simulink model "micro_hydro_with_elc"  (R2018a)
settings: Solver=ode23tb  StartTime=0.0  StopTime=4  FixedStep=1e-6  RelTol=1e-3
libraries: powerlib x37, powerlib_meascontrol x9, simulink x1, sps_avr x1, spsHTGModel x1
settings Model: SimulationMode=accelerator  Creator=deep  LastModifiedBy=Electrical
settings SolverCC: AlgebraicLoopSolver=LineSearch
settings OptimizationCC: EfficientMapNaN2IntZero=off
settings HardwareCC: TargetBitPerPointer=64  TargetBitPerSizeT=64  TargetBitPerPtrDiffT=64  TargetLongLongMode=on  TargetIntDivRoundTo=Zero  TargetEndianess=LittleEndian  TargetWordSize=64  TargetHWDeviceType=MATLAB Host  ProdEqTarget=off
settings SFSimCC: SimUseLocalCustomCode=on
settings RTWCC: RTWUseLocalCustomCode=on
settings CodeAppCC: MaxIdLength=128
settings GRTTargetCC: TargetLangStandard=C89/C90 (ANSI)  CombineOutputUpdateFcns=off  GRTInterface=on

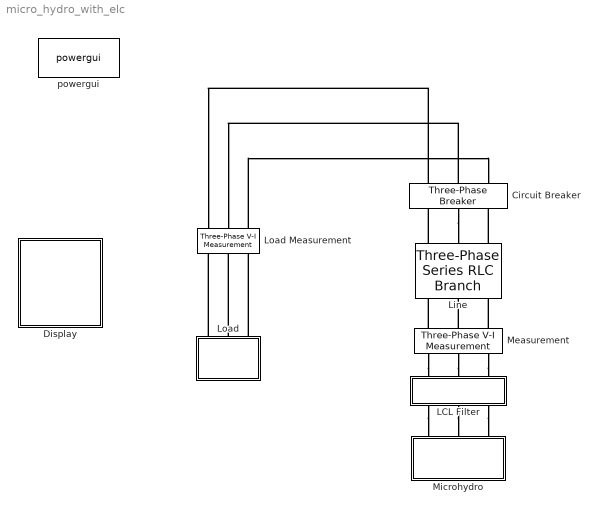
== system micro_hydro_with_elc ==
  Circuit Breaker : powerlib/Elements/Three-Phase Breaker  InitialState=open  SwitchA=on  SwitchB=on  SwitchC=on  SwitchTimes=[0.5 4]  External=off  BreakerResistance=0.00001  SnubberResistance=500000  SnubberCapacitance=inf  Measurements=None
  Display : Subsystem
  LCL Filter : Subsystem  mask{L=0.5e-3, C=100e-6}
      mask prompts: L "Inductance(L)"; C "Capacitance(C)"
  Line : powerlib/Elements/Three-Phase Series RLC Branch  LConnTagsString=A|B|C  RConnTagsString=A|B|C  BranchType=RL  Resistance=1  Inductance=0.0125  Capacitance=0  Measurements=None
  Load : Subsystem
  Load Measurement : powerlib/Measurements/Three-Phase V-I Measurement  VoltageMeasurement=phase-to-ground  SetLabelV=on  LabelV=Vload  Vpu=off  VpuLL=off  CurrentMeasurement=yes  SetLabelI=on  LabelI=Iload  Ipu=off  Pbase=100e6  Vbase=500e3  OutputType=Complex  PhasorSimulation=off  PSBequivalent=0
  Measurement : powerlib/Measurements/Three-Phase V-I Measurement  VoltageMeasurement=phase-to-ground  SetLabelV=on  LabelV=Vgrid  Vpu=off  VpuLL=off  CurrentMeasurement=yes  SetLabelI=on  LabelI=Igrid  Ipu=off  Pbase=100e6  Vbase=500e3  OutputType=Complex  PhasorSimulation=off  PSBequivalent=0
  Microhydro : Subsystem
  powergui : powerlib/powergui  Priority=1  SimulationMode=Discrete  SampleTime=1e-6  frequency=60  Iterations=50  frequencyindice=0  Pbase=100e6  ErrMax=1e-4  UnitsV=kV  UnitsW=MW  buscounter=0  FunctionMessages=off  echomessages=off  EnableUseOfTLC=off  CurrentSourceSwitches=off  DisableSnubberDevices=off  DisableRonSwitches=off  DisableVfSwitches=off  DisplayEquations=off  SolverType=Tustin/Backward Euler (TBE)  Interpol=off  ExternalGateDelay=off  methode=off  Ts=100  x0status=zero  SPID=off  SwTol=0  HookPort=off  RestoreLinks=warning  ResistiveCurrentMeasurement=off  Frange=[0:2:500]  Ylog=off  Xlog=on  ShowGrid=off  save=off  variable=ZData  structure=logsout  ZoomFFT=off  StartTime=0.0  cycles=1  DisplayStyle=1  fundamental=60  FreqAxis=off  MaxFrequency=1000  frequencyindicesteady=1  RmsSteady=1  display=off
  connections:
  Circuit Breaker/RConn1 -- Load Measurement/LConn1
  Load Measurement/LConn3 -- Circuit Breaker/RConn3
  LCL Filter/LConn2 -- Microhydro/RConn2
  LCL Filter/LConn3 -- Microhydro/RConn3
  LCL Filter/LConn1 -- Microhydro/RConn1
  Circuit Breaker/RConn2 -- Load Measurement/LConn2
  Line/RConn1 -- Circuit Breaker/LConn1
  Circuit Breaker/LConn2 -- Line/RConn2
  Line/RConn3 -- Circuit Breaker/LConn3
  Measurement/RConn1 -- Line/LConn1
  Measurement/RConn2 -- Line/LConn2
  Measurement/RConn3 -- Line/LConn3
  Measurement/LConn1 -- LCL Filter/RConn1
  Measurement/LConn2 -- LCL Filter/RConn2
  Measurement/LConn3 -- LCL Filter/RConn3
  Load/LConn1 -- Load Measurement/RConn1
  Load/LConn2 -- Load Measurement/RConn2
  Load/LConn3 -- Load Measurement/RConn3

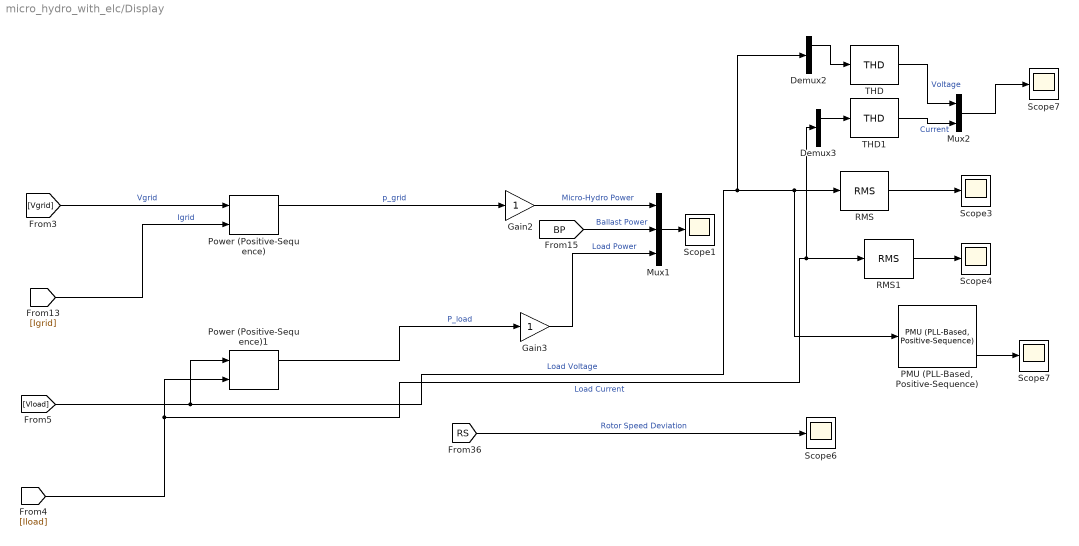
== system micro_hydro_with_elc/Display ==
  Demux2 : Demux  Outputs=3
  Demux3 : Demux  Outputs=3
  Gain2 : Gain
  Gain3 : Gain
  Mux1 : Mux  Inputs=3
  Mux2 : Mux  Inputs=2
  "PMU (PLL-Based, Positive-Sequence)" : powerlib_meascontrol/Measurements/PMU (PLL-Based, Positive-Sequence)  nominalFrequency=50  samplingRate=64  reportingFactor=1
      settings: SourceProductName=Simscape Power Systems  SourceProductBaseCode=PS
  Power (Positive-Sequence) : powerlib_meascontrol/Measurements/Power (Positive-Sequence)  Freq=50  Vinit=[0, 0]  Iinit=[0, 0]  Ts=0
      settings: SourceProductName=Simscape Power Systems  SourceProductBaseCode=PS
  Power (Positive-Sequence)1 : powerlib_meascontrol/Measurements/Power (Positive-Sequence)  Freq=50  Vinit=[0, 0]  Iinit=[0, 0]  Ts=0
      settings: SourceProductName=Simscape Power Systems  SourceProductBaseCode=PS
  RMS : powerlib_meascontrol/Measurements/RMS  TrueRMS=on  Freq=50  RMSInit=0  Ts=0
  RMS1 : powerlib_meascontrol/Measurements/RMS  TrueRMS=on  Freq=50  RMSInit=0  Ts=0
  Scope{1,3..4,6..7} (5 alike) : Scope
  "Scope7 " : Scope
  THD : powerlib_meascontrol/Measurements/THD  Freq=50  Ts=0
  THD1 : powerlib_meascontrol/Measurements/THD  Freq=50  Ts=0
  wires:
  Power (Positive-Sequence)/1 -> Gain2/1  "p_grid"
  [Vgrid] -> Power (Positive-Sequence)/1  "Vgrid"
  [Iload] -> Power (Positive-Sequence)1/2, Demux3/1, RMS1/1  "Load Current"
  Power (Positive-Sequence)1/1 -> Gain3/1  "P_load"
  [RS] -> Scope6/1  "Rotor Speed Deviation"
  [Vload] -> Power (Positive-Sequence)1/1, Demux2/1, "PMU (PLL-Based, Positive-Sequence)"/1, RMS/1  "Load Voltage"
  Mux1/1 -> Scope1/1
  RMS/1 -> Scope3/1
  RMS1/1 -> Scope4/1
  "PMU (PLL-Based, Positive-Sequence)"/3 -> Scope7/1
  Demux2/1 -> THD/1
  Demux3/1 -> THD1/1
  THD/1 -> Mux2/1  "Voltage"
  THD1/1 -> Mux2/2  "Current"
  Mux2/1 -> "Scope7 "/1
  Gain2/1 -> Mux1/1  "Micro-Hydro Power"
  [BP] -> Mux1/2  "Ballast Power"
  Gain3/1 -> Mux1/3  "Load Power"
  [Igrid] -> Power (Positive-Sequence)/2  "Igrid"

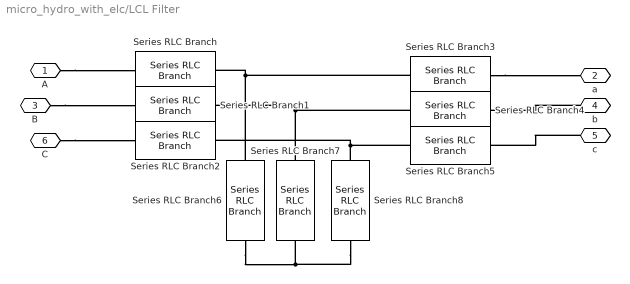
== system micro_hydro_with_elc/LCL Filter ==
  Series RLC Branch{,1..5} (6 alike) : powerlib/Elements/Series RLC Branch  LConnTagsString=__new0  RConnTagsString=__new0  BranchType=L  Resistance=1  Inductance=L  SetiL0=off  InitialCurrent=0  Capacitance=1e-6  Setx0=off  InitialVoltage=0  Measurements=None
  Series RLC Branch6 : powerlib/Elements/Series RLC Branch  LConnTagsString=__new0  RConnTagsString=__new0  BranchType=C  Resistance=1  Inductance=0.5e-3  SetiL0=off  InitialCurrent=0  Capacitance=C  Setx0=off  InitialVoltage=0  Measurements=None
  Series RLC Branch7 : powerlib/Elements/Series RLC Branch  LConnTagsString=__new0  RConnTagsString=__new0  BranchType=C  Resistance=1  Inductance=0.5e-3  SetiL0=off  InitialCurrent=0  Capacitance=C  Setx0=off  InitialVoltage=0  Measurements=None
  Series RLC Branch8 : powerlib/Elements/Series RLC Branch  LConnTagsString=__new0  RConnTagsString=__new0  BranchType=C  Resistance=1  Inductance=0.5e-3  SetiL0=off  InitialCurrent=0  Capacitance=C  Setx0=off  InitialVoltage=0  Measurements=None
  A : PMIOPort  Side=Left
  a : PMIOPort  Port=2  Side=Right
  B : PMIOPort  Port=3  Side=Left
  b : PMIOPort  Port=4  Side=Right
  c : PMIOPort  Port=5  Side=Right
  C : PMIOPort  Port=6  Side=Left
  connections:
  C/RConn1 -- Series RLC Branch2/LConn1
  Series RLC Branch3/LConn1 -- Series RLC Branch/RConn1 -- Series RLC Branch6/LConn1
  Series RLC Branch3/RConn1 -- a/RConn1
  Series RLC Branch6/RConn1 -- Series RLC Branch8/RConn1 -- Series RLC Branch7/RConn1
  Series RLC Branch5/LConn1 -- Series RLC Branch2/RConn1 -- Series RLC Branch8/LConn1
  Series RLC Branch4/LConn1 -- Series RLC Branch1/RConn1 -- Series RLC Branch7/LConn1
  c/RConn1 -- Series RLC Branch5/RConn1
  A/RConn1 -- Series RLC Branch/LConn1
  B/RConn1 -- Series RLC Branch1/LConn1
  b/RConn1 -- Series RLC Branch4/RConn1

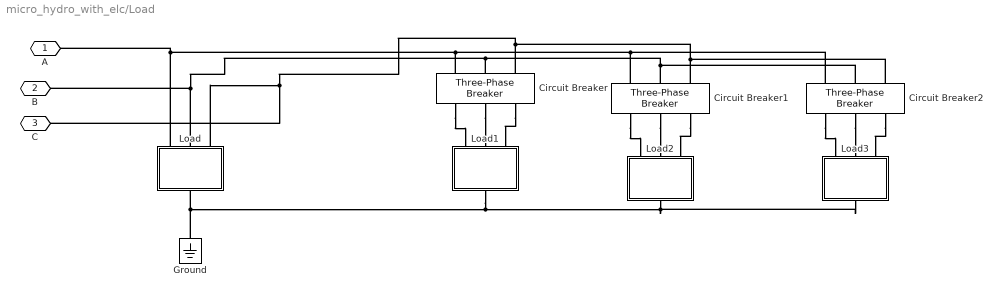
== system micro_hydro_with_elc/Load ==
  Circuit Breaker : powerlib/Elements/Three-Phase Breaker  InitialState=open  SwitchA=on  SwitchB=on  SwitchC=on  SwitchTimes=[1.5 4]  External=off  BreakerResistance=0.00001  SnubberResistance=500000  SnubberCapacitance=inf  Measurements=None
  Circuit Breaker1 : powerlib/Elements/Three-Phase Breaker  InitialState=open  SwitchA=on  SwitchB=on  SwitchC=on  SwitchTimes=[2.5 4]  External=off  BreakerResistance=0.00001  SnubberResistance=500000  SnubberCapacitance=inf  Measurements=None
  Circuit Breaker2 : powerlib/Elements/Three-Phase Breaker  InitialState=open  SwitchA=on  SwitchB=on  SwitchC=on  SwitchTimes=[3.5 4]  External=off  BreakerResistance=0.00001  SnubberResistance=500000  SnubberCapacitance=inf  Measurements=None
  Ground : powerlib/Elements/Ground  LConnTagsString=a
  Load : Subsystem  mask{R=100}
      mask prompts: R "Load Resistance"
      mask DialogControl DescTextVar Prompt: Load in terms of Resistance
  Load1 : Subsystem  mask{R=100}
      mask prompts: R "Load Resistance"
      mask DialogControl DescTextVar Prompt: Load in terms of Resistance
  Load2 : Subsystem  mask{R=100}
      mask prompts: R "Load Resistance"
      mask DialogControl DescTextVar Prompt: Load in terms of Resistance
  Load3 : Subsystem  mask{R=100}
      mask prompts: R "Load Resistance"
      mask DialogControl DescTextVar Prompt: Load in terms of Resistance
  A : PMIOPort  Side=Left
  B : PMIOPort  Port=2  Side=Left
  C : PMIOPort  Port=3  Side=Left
  connections:
  Ground/LConn1 -- Load3/RConn1 -- Load2/RConn1 -- Load1/RConn1 -- Load/RConn1
  Load/LConn1 -- Circuit Breaker2/RConn1 -- Circuit Breaker1/RConn1 -- Circuit Breaker/RConn1 -- A/RConn1
  Load/LConn2 -- Circuit Breaker2/RConn2 -- Circuit Breaker1/RConn2 -- Circuit Breaker/RConn2 -- B/RConn1
  Load/LConn3 -- Circuit Breaker2/RConn3 -- Circuit Breaker1/RConn3 -- Circuit Breaker/RConn3 -- C/RConn1
  Circuit Breaker/LConn2 -- Load1/LConn2
  Circuit Breaker/LConn1 -- Load1/LConn1
  Circuit Breaker/LConn3 -- Load1/LConn3
  Circuit Breaker1/LConn2 -- Load2/LConn2
  Circuit Breaker1/LConn1 -- Load2/LConn1
  Circuit Breaker1/LConn3 -- Load2/LConn3
  Circuit Breaker2/LConn2 -- Load3/LConn2
  Circuit Breaker2/LConn1 -- Load3/LConn1
  Circuit Breaker2/LConn3 -- Load3/LConn3

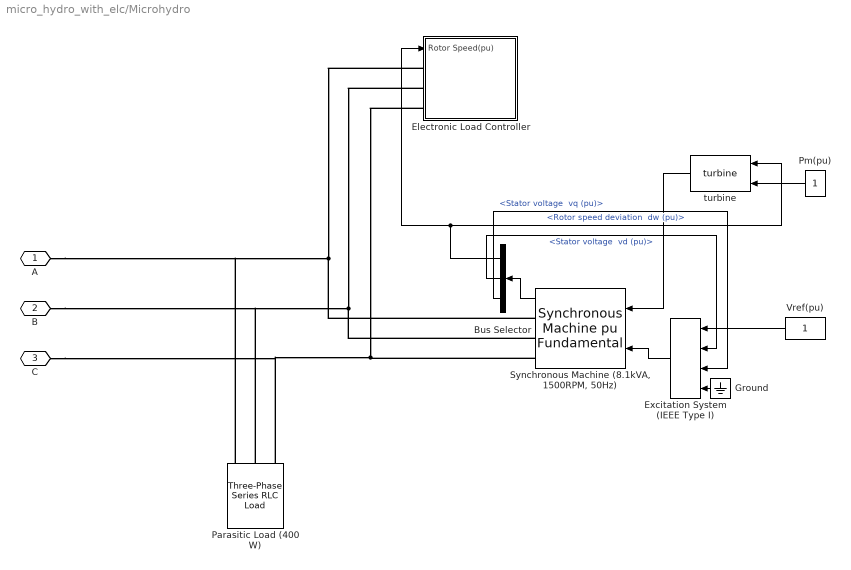
== system micro_hydro_with_elc/Microhydro ==
  Bus Selector : BusSelector  OutputSignals="Mechanical.Rotor speed deviation  dw (pu),dq0 components.Stator voltage  vd (pu),dq0 components.Stator voltage  vq (pu)"
  Electronic Load Controller : Subsystem
  Excitation System (IEEE Type I) : sps_avr/Excitation System  tr=20e-3  reg=[ 300, 0.001 ]  exc=[ 1, 0 ]  tgr=[ 0, 0 ]  damp=[ 0.001, 0.1 ]  sat=[ 0, 0 ]  lim=[ -11.5, 11.5, 0 ]  v0="[1.0  1.28]"
      settings: SourceProductName=Simscape Power Systems  SourceProductBaseCode=PS
  Ground : Ground
  Parasitic Load (400 W) : powerlib/Elements/Three-Phase Series RLC Load  LConnTagsString=A|B|C  Configuration=Y (grounded)  NominalVoltage=400  Vabc=[1e3 1e3 1e3]  Vabcp=[1e3 1e3 1e3]  NominalFrequency=50  UnbalancedPower=off  ActivePower=400  InductivePower=0  CapacitivePower=0  Pabc=[10e3 9e3 11e3]  QLabc=[100 90 110]  QCabc=[100 90 110]  Pabcp=[10e3 9e3 11e3]  QLabcp=[100 90 110]  QCabcp=[100 90 110]  Measurements=None  LoadType=constant Z
  Pm(pu) : Constant  SampleTime=-1
  "Synchronous Machine (8.1kVA, 1500RPM, 50Hz)" : powerlib/Machines/Synchronous Machine pu Fundamental  PresetModel=01: 50Hz 400V 8.1kVA 1500RPM  MechanicalLoad=Mechanical power Pm  ShowDetailedParameters=on  RotorType=Salient-pole  Units=per unit fundamental parameters  MeasurementBus=off  NominalParameters=[8100 400 50]  Stator=[0.08201 0.072 1.728 0.823]  Field=[0.06117 0.1801]  Dampers2=[0.0652, 0.5134, 0.0287, 0.2553, 7.765e-3, 0.9167 ]  Dampers1=[0.1591 0.1166 0.2416 0.1615]  Mechanical=[0.1406 0.02742 2]  PolePairs=2  InitialConditions="[ 0  0  0  0  0  0  -120  -240  1 ]"  SetSaturation=off  Saturation=[0.6404,0.7127,0.8441,0.9214,0.9956,1.082,1.19,1.316,1.457;0.7,0.7698,0.8872,0.9466,0.9969,1.046,1.1,1.151,1.201]  LoadFlowParameters=[1,0,0,0,0]  TsPowergui=0  TsBlock=-1  IterativeModel=Trapezoidal non iterative  IterativeDiscreteModel=Trapezoidal non iterative  BusType=PV  Pref=8100  Qref=0  Qmin=-inf  Qmax=inf  PLF=0  QLF=0
      settings: SourceProductName=Simscape Power Systems  SourceProductBaseCode=PS
  Vref(pu) : Constant  SampleTime=-1
  turbine : spsHTGModel/Discrete/turbine  SystemSampleTime=-1
      link override Gain2: Gain=1/1
      link override beta: Gain=1
      link override position: InitialCondition=1
      link override turbine gain: Gain=1
  A : PMIOPort  Side=Right
  B : PMIOPort  Port=2  Side=Right
  C : PMIOPort  Port=3  Side=Right
  wires:
  Bus Selector/1 -> turbine/1, Electronic Load Controller/1(Rotor Speed(pu))  "<Rotor speed deviation  dw (pu)>"
  "Synchronous Machine (8.1kVA, 1500RPM, 50Hz)"/1 -> Bus Selector/1
  Excitation System (IEEE Type I)/1 -> "Synchronous Machine (8.1kVA, 1500RPM, 50Hz)"/2
  Bus Selector/2 -> Excitation System (IEEE Type I)/2  "<Stator voltage  vd (pu)>"
  Bus Selector/3 -> Excitation System (IEEE Type I)/3  "<Stator voltage  vq (pu)>"
  Ground/1 -> Excitation System (IEEE Type I)/4
  Pm(pu)/1 -> turbine/2
  turbine/1 -> "Synchronous Machine (8.1kVA, 1500RPM, 50Hz)"/1
  Vref(pu)/1 -> Excitation System (IEEE Type I)/1
  connections:
  Electronic Load Controller/LConn2 -- B/RConn1 -- Parasitic Load (400 W)/LConn2 -- "Synchronous Machine (8.1kVA, 1500RPM, 50Hz)"/RConn2
  Electronic Load Controller/LConn1 -- A/RConn1 -- Parasitic Load (400 W)/LConn1 -- "Synchronous Machine (8.1kVA, 1500RPM, 50Hz)"/RConn1
  Electronic Load Controller/LConn3 -- Parasitic Load (400 W)/LConn3 -- C/RConn1 -- "Synchronous Machine (8.1kVA, 1500RPM, 50Hz)"/RConn3

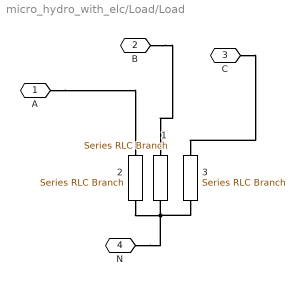
== system micro_hydro_with_elc/Load/Load ==
  1 : powerlib/Elements/Series RLC Branch  LConnTagsString=__new0  RConnTagsString=__new0  BranchType=R  Resistance=R  Inductance=10e-3  SetiL0=off  InitialCurrent=0  Capacitance=1e-6  Setx0=off  InitialVoltage=0  Measurements=None
  2 : powerlib/Elements/Series RLC Branch  LConnTagsString=__new0  RConnTagsString=__new0  BranchType=R  Resistance=R  Inductance=10e-3  SetiL0=off  InitialCurrent=0  Capacitance=1e-6  Setx0=off  InitialVoltage=0  Measurements=None
  3 : powerlib/Elements/Series RLC Branch  LConnTagsString=__new0  RConnTagsString=__new0  BranchType=R  Resistance=R  Inductance=10e-3  SetiL0=off  InitialCurrent=0  Capacitance=1e-6  Setx0=off  InitialVoltage=0  Measurements=None
  A : PMIOPort  Side=Left
  B : PMIOPort  Port=2  Side=Left
  C : PMIOPort  Port=3  Side=Left
  N : PMIOPort  Port=4  Side=Right
  connections:
  A/RConn1 -- 2/LConn1
  B/RConn1 -- 1/LConn1
  C/RConn1 -- 3/LConn1
  1/RConn1 -- 3/RConn1 -- N/RConn1 -- 2/RConn1

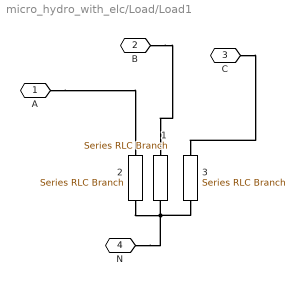
== system micro_hydro_with_elc/Load/Load1 ==
  1 : powerlib/Elements/Series RLC Branch  LConnTagsString=__new0  RConnTagsString=__new0  BranchType=R  Resistance=R  Inductance=10e-3  SetiL0=off  InitialCurrent=0  Capacitance=1e-6  Setx0=off  InitialVoltage=0  Measurements=None
  2 : powerlib/Elements/Series RLC Branch  LConnTagsString=__new0  RConnTagsString=__new0  BranchType=R  Resistance=R  Inductance=10e-3  SetiL0=off  InitialCurrent=0  Capacitance=1e-6  Setx0=off  InitialVoltage=0  Measurements=None
  3 : powerlib/Elements/Series RLC Branch  LConnTagsString=__new0  RConnTagsString=__new0  BranchType=R  Resistance=R  Inductance=10e-3  SetiL0=off  InitialCurrent=0  Capacitance=1e-6  Setx0=off  InitialVoltage=0  Measurements=None
  A : PMIOPort  Side=Left
  B : PMIOPort  Port=2  Side=Left
  C : PMIOPort  Port=3  Side=Left
  N : PMIOPort  Port=4  Side=Right
  connections:
  A/RConn1 -- 2/LConn1
  B/RConn1 -- 1/LConn1
  C/RConn1 -- 3/LConn1
  1/RConn1 -- 3/RConn1 -- N/RConn1 -- 2/RConn1

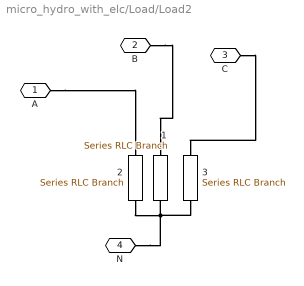
== system micro_hydro_with_elc/Load/Load2 ==
  1 : powerlib/Elements/Series RLC Branch  LConnTagsString=__new0  RConnTagsString=__new0  BranchType=R  Resistance=R  Inductance=10e-3  SetiL0=off  InitialCurrent=0  Capacitance=1e-6  Setx0=off  InitialVoltage=0  Measurements=None
  2 : powerlib/Elements/Series RLC Branch  LConnTagsString=__new0  RConnTagsString=__new0  BranchType=R  Resistance=R  Inductance=10e-3  SetiL0=off  InitialCurrent=0  Capacitance=1e-6  Setx0=off  InitialVoltage=0  Measurements=None
  3 : powerlib/Elements/Series RLC Branch  LConnTagsString=__new0  RConnTagsString=__new0  BranchType=R  Resistance=R  Inductance=10e-3  SetiL0=off  InitialCurrent=0  Capacitance=1e-6  Setx0=off  InitialVoltage=0  Measurements=None
  A : PMIOPort  Side=Left
  B : PMIOPort  Port=2  Side=Left
  C : PMIOPort  Port=3  Side=Left
  N : PMIOPort  Port=4  Side=Right
  connections:
  A/RConn1 -- 2/LConn1
  B/RConn1 -- 1/LConn1
  C/RConn1 -- 3/LConn1
  1/RConn1 -- 3/RConn1 -- N/RConn1 -- 2/RConn1

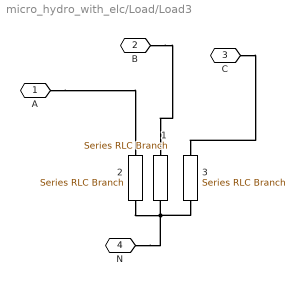
== system micro_hydro_with_elc/Load/Load3 ==
  1 : powerlib/Elements/Series RLC Branch  LConnTagsString=__new0  RConnTagsString=__new0  BranchType=R  Resistance=R  Inductance=10e-3  SetiL0=off  InitialCurrent=0  Capacitance=1e-6  Setx0=off  InitialVoltage=0  Measurements=None
  2 : powerlib/Elements/Series RLC Branch  LConnTagsString=__new0  RConnTagsString=__new0  BranchType=R  Resistance=R  Inductance=10e-3  SetiL0=off  InitialCurrent=0  Capacitance=1e-6  Setx0=off  InitialVoltage=0  Measurements=None
  3 : powerlib/Elements/Series RLC Branch  LConnTagsString=__new0  RConnTagsString=__new0  BranchType=R  Resistance=R  Inductance=10e-3  SetiL0=off  InitialCurrent=0  Capacitance=1e-6  Setx0=off  InitialVoltage=0  Measurements=None
  A : PMIOPort  Side=Left
  B : PMIOPort  Port=2  Side=Left
  C : PMIOPort  Port=3  Side=Left
  N : PMIOPort  Port=4  Side=Right
  connections:
  A/RConn1 -- 2/LConn1
  B/RConn1 -- 1/LConn1
  C/RConn1 -- 3/LConn1
  1/RConn1 -- 3/RConn1 -- N/RConn1 -- 2/RConn1

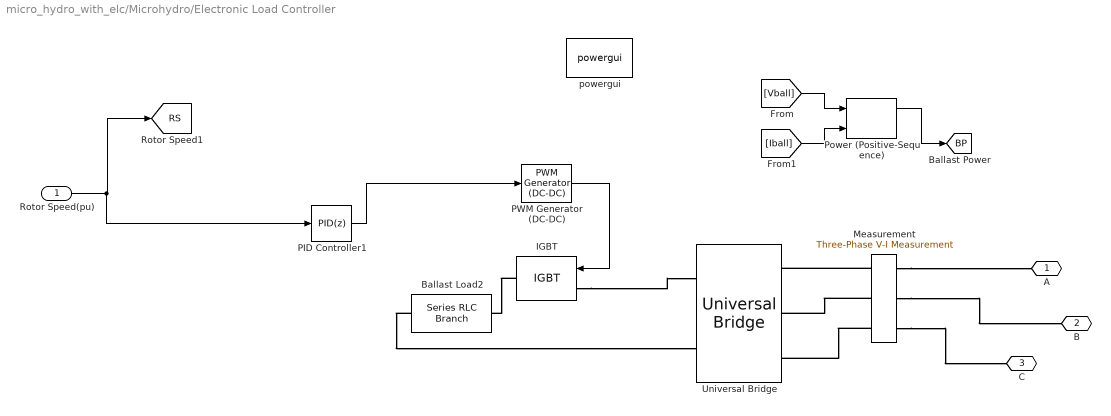
== system micro_hydro_with_elc/Microhydro/Electronic Load Controller ==
  Rotor Speed(pu) : Inport
  Ballast Load2 : powerlib/Elements/Series RLC Branch  LConnTagsString=__new0  RConnTagsString=__new0  BranchType=R  Resistance=10  Inductance=10e-3  SetiL0=off  InitialCurrent=0  Capacitance=1e-6  Setx0=off  InitialVoltage=0  Measurements=None
  IGBT : powerlib/Power Electronics/IGBT  Ron=0.001  Lon=0  Vf=1  Tf=1e-6  Tt=2e-6  IC=0  Rs=1e8  Cs=inf  Measurements=off
  Measurement : powerlib/Measurements/Three-Phase V-I Measurement  VoltageMeasurement=phase-to-ground  SetLabelV=on  LabelV=Vball  Vpu=off  VpuLL=off  CurrentMeasurement=yes  SetLabelI=on  LabelI=Iball  Ipu=off  Pbase=100e6  Vbase=500e3  OutputType=Complex  PhasorSimulation=off  PSBequivalent=0
  PID Controller1 : simulink/Continuous/PID Controller  Controller=PID  TimeDomain=Discrete-time  SampleTime=1e-6  IntegratorMethod=Forward Euler  FilterMethod=Forward Euler  Form=Ideal  UseFilter=off  ControllerParametersSource=internal  P=50  I=100  D=0.05  N=100  InitialConditionSource=internal  InitialConditionForIntegrator=0  InitialConditionForFilter=0  ExternalReset=none  ZeroCross=off  LimitOutput=on  UpperSaturationLimit=1  LowerSaturationLimit=0  LinearizeAsGain=on  AntiWindupMode=none  Kb=1  TrackingMode=off  Kt=1  PParamMin=[]  PParamMax=[]  IParamMin=[]  IParamMax=[]  DParamMin=[]  DParamMax=[]  NParamMin=[]  NParamMax=[]  KbParamMin=[]  KbParamMax=[]  KtParamMin=[]  KtParamMax=[]  POutMin=[]  POutMax=[]  IOutMin=[]  IOutMax=[]  DOutMin=[]  DOutMax=[]  NOutMin=[]  NOutMax=[]  KbOutMin=[]  KbOutMax=[]  KtOutMin=[]  KtOutMax=[]  IntegratorOutMin=[]  IntegratorOutMax=[]  FilterOutMin=[]  FilterOutMax=[]  SumOutMin=[]  SumOutMax=[]  SumI1OutMin=[]  SumI1OutMax=[]  SumI2OutMin=[]  SumI2OutMax=[]  SumI3OutMin=[]  SumI3OutMax=[]  SumDOutMin=[]  SumDOutMax=[]  SaturationOutMin=[]  SaturationOutMax=[]  IntegratorContinuousStateAttributes=''  IntegratorStateMustResolveToSignalObject=off  IntegratorRTWStateStorageClass=Auto  FilterContinuousStateAttributes=''  FilterStateMustResolveToSignalObject=off  FilterRTWStateStorageClass=Auto  DifferentiatorICPrevScaledInput=0  DifferentiatorOutMin=[]  DifferentiatorOutMax=[]  FilterDiffOutCoefMin=[]  FilterDiffOutCoefMax=[]  SumDenOutMin=[]  SumDenOutMax=[]  SumNumOutMin=[]  SumNumOutMax=[]  ReciprocalOutMin=[]  ReciprocalOutMax=[]  DivideOutMin=[]  DivideOutMax=[]  TunerSelectOption=Transfer Function Based (PID Tuner App)
  PWM Generator (DC-DC) : powerlib_meascontrol/Pulse & Signal Generators/PWM Generator (DC-DC)  Fsw=4000  Ts=1e-6
  Power (Positive-Sequence) : powerlib_meascontrol/Measurements/Power (Positive-Sequence)  Freq=50  Vinit=[0, 0]  Iinit=[0, 0]  Ts=0
      settings: SourceProductName=Simscape Power Systems  SourceProductBaseCode=PS
  Universal Bridge : powerlib/Power Electronics/Universal Bridge  Arms=3  SnubberResistance=1e6  SnubberCapacitance=10e-9  Device=Diodes  Ron=1e-3  Lon=0  ForwardVoltages="[  0  0  ]"  ForwardVoltage=0  GTOparameters=[ 10e-6 , 20e-6 ]  IGBTparameters=[ 1e-6 , 2e-6 ]  Measurements=None  Measurements_2=None  converterType=Rectifier
  powergui : powerlib/powergui  Priority=1  SimulationMode=Discrete  SampleTime=1e-6  frequency=50  Iterations=50  frequencyindice=0  Pbase=100e6  ErrMax=1e-4  UnitsV=kV  UnitsW=MW  buscounter=0  FunctionMessages=off  echomessages=off  EnableUseOfTLC=off  CurrentSourceSwitches=off  DisableSnubberDevices=off  DisableRonSwitches=off  DisableVfSwitches=off  DisplayEquations=off  SolverType=Tustin/Backward Euler (TBE)  Interpol=off  ExternalGateDelay=off  methode=off  Ts=100  x0status=zero  SPID=off  SwTol=0  HookPort=off  RestoreLinks=warning  ResistiveCurrentMeasurement=off  Frange=[0:2:500]  Ylog=off  Xlog=on  ShowGrid=off  save=off  variable=ZData  structure=Source_Current  ZoomFFT=on  StartTime=1.295  cycles=10  DisplayStyle=1  fundamental=50  FreqAxis=off  MaxFrequency=1000  frequencyindicesteady=1  RmsSteady=1  display=off
  A : PMIOPort  Side=Left
  B : PMIOPort  Port=2  Side=Left
  C : PMIOPort  Port=3  Side=Left
  tag scope: BP=global, RS=global
  wires:
  PID Controller1/1 -> PWM Generator (DC-DC)/1
  PWM Generator (DC-DC)/1 -> IGBT/1
  Rotor Speed(pu)/1 -> PID Controller1/1, [RS]
  [Vball] -> Power (Positive-Sequence)/1
  [Iball] -> Power (Positive-Sequence)/2
  Power (Positive-Sequence)/1 -> [BP]
  connections:
  Ballast Load2/RConn1 -- Universal Bridge/RConn2
  IGBT/LConn1 -- Universal Bridge/RConn1
  IGBT/RConn1 -- Ballast Load2/LConn1
  Measurement/RConn1 -- Universal Bridge/LConn1
  Measurement/RConn2 -- Universal Bridge/LConn2
  Measurement/RConn3 -- Universal Bridge/LConn3
  Measurement/LConn1 -- A/RConn1
  Measurement/LConn2 -- B/RConn1
  Measurement/LConn3 -- C/RConn1
